simulink model "mrsDiffDrivePathFollowingModel"  (R2023a)
settings: Solver=VariableStepAuto  StartTime=0.0  StopTime=42  FixedStep=0.01  RelTol=1e-3  EnableMultiTasking=on
PreLoadFcn:
  | % Simulation parameters
  | sampleTime = 0.1;
  | 
  | % Vehicle parameters
  | R = 0.1;
  | L = 0.5;
  | 
  | % Lidar parameters
  | load exampleMap
  | scanAngles = linspace(-pi/2,pi/2,51);
  | scanMaxRange = 5;
  | scanSensorOffset = [0,0];
libraries: mobileRoboticsLib x4, simulink x2, robotalgslib x2
settings Model: Creator=scastro  LastModifiedBy=John_117
settings SolverCC: AlgebraicLoopSolver=TrustRegion
settings DataIOCC: LimitDataPoints=on  ReturnWorkspaceOutputs=off
settings OptimizationCC: LifeSpan=inf
settings DebuggingCC: UnconnectedInputMsg=warning  UnconnectedOutputMsg=warning  UnconnectedLineMsg=warning  AllowSymbolicDim=off  SFUnexpectedBacktrackingDiag=warning  SFNoUnconditionalDefaultTransitionDiag=warning  SFExecutionAtInitializationDiag=none  ArithmeticOperatorsInVariantConditions=warning
settings ModelReferenceCC: EnableRefExpFcnMdlSchedulingChecks=on
settings SFSimCC: SimUseLocalCustomCode=off  CustomCodeUndefinedFunction=UseInterfaceOnly
settings RTWCC: RTWUseLocalCustomCode=off
settings CodeAppCC: StateflowObjectComments=on
settings GRTTargetCC: TargetLangStandard=C89/C90 (ANSI)
settings ConfigComp: CovMetricSettings=dw  CovSaveCumulativeToWorkspaceVar=on  CovSaveSingleToWorkspaceVar=on  CovExternalEMLEnable=off  CovSFcnEnable=off
settings SimscapeCC: SimscapeNominalValues="[{\"value\":\"10\",\"unit\":\"V\"},{\"value\":\"1\",\"unit\":\"A\"},{\"value\":\"10\",\"unit\":\"N*m\"},{\"value\":\"10\",\"unit\":\"bar\"},{\"value\":\"100\",\"unit\":\"kJ/kg\"},{\"value\":\"1\",\"unit\":\"kW\"},{\"value\":\"300\",\"unit\":\"K\"},{\"value\":\"100\",\"unit\":\"cm^3/s\"},{\"value\":\"1\",\"unit\":\"kN\"},{\"value\":\"1\",\"unit\":\"g/cm^3\"},{\"value\":\"1\",\"unit\":\"l\"},{\"value\":\"1\",\"unit\":\"cm^2\"},{\"value\":\"60\",\"unit\":\"Hz\"}]"  SimscapeLogType=all  SimscapeLogDataHistory=10000
settings ConfigurationSet: Description=SimMechanics 2G
settings ExplorerConfigSet: InternalSimMechanicsExplorerSettings="<ExplorerConfiguration><canonicalview>default</canonicalview><AnimationSetting><BasePlaybackSpeed>1.0</BasePlaybackSpeed><PlaybackSpeedFactor>1.0</PlaybackSpeedFactor></AnimationSetting><TilePanel><TileInfo><Tiles Columns=\"1\" Count=\"1\" Rows=\"1\"><Column Weight=\"1\"/><Row Weight=\"1\"/><Tile Height=\"1\" Width=\"1\" X=\"0\" Y=\"0\"/></Tiles></TileInfo><SceneInfo><SceneViewer><BGColor><R>0.60000002384185791</R><G>0.60000002384185791</G><B>0.60000002384185791</B></BGColor><Camera><DoPerspective>off</DoPerspective><Position><X>-1.70656042355848525</X><Y>-0.974920623359631922</Y><Z>4.72930454537082046</Z></Position><Center><X>0.552860638431633689</X><Y>1.42025063411503494</Y><Z>1.4843509506914252</Z></Center><Up><X>0.664249622453917166</X><Y>0.300615402055903091</Y><Z>0.684399604848363485</Z></Up><ViewLimDist>1</ViewLimDist><YLim>2.77881717169207398</YLim><XLim>3.55928742670435394</XLim></Camera></SceneViewer></SceneInfo></TilePanel><MechEditorPanel><Cameras/><GfxPanelCameraMap/><VideoCreator><PlaybackSpeedRatio>1.0</PlaybackSpeedRatio><FrameRate>30</FrameRate><VideoFormat>Motion JPEG AVI</VideoFormat><FrameSize>auto</FrameSize></VideoCreator></MechEditorPanel></ExplorerConfiguration>"

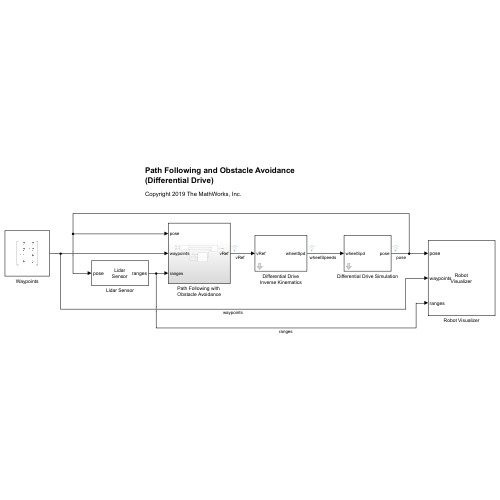
[thumbnail: Simulink's stored preview of the top-level diagram]
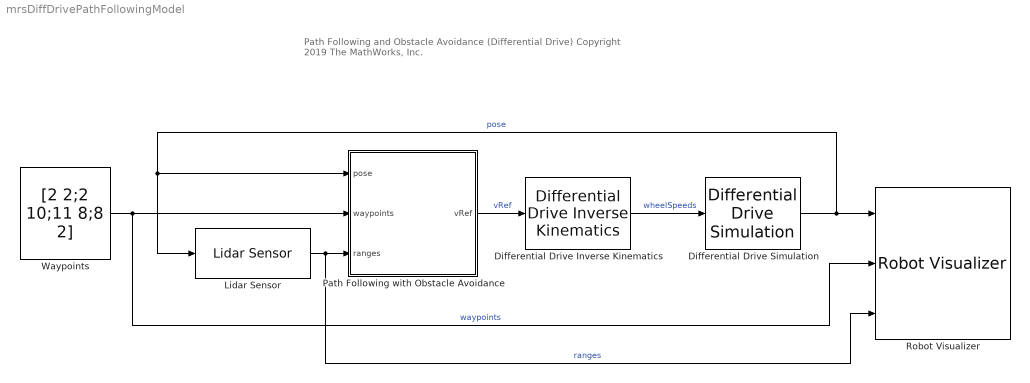
== system mrsDiffDrivePathFollowingModel ==
  note: Path Following and Obstacle Avoidance
      | (Differential Drive)
      |
      | Copyright 2019 The MathWorks, Inc.
  Differential Drive Inverse Kinematics : mobileRoboticsLib/Kinematic Models/Differential Drive/Differential Drive Inverse Kinematics  wheelRadius=R  wheelBase=L
      settings: SourceProductName=Mobile Robotics Simulation Toolbox
  Differential Drive Simulation : mobileRoboticsLib/Kinematic Models/Differential Drive/Differential Drive Simulation  wheelRadius=R  wheelBase=L  initX=2  initY=2  initAngle=0  Ts=sampleTime
      settings: SourceProductName=Mobile Robotics Simulation Toolbox
  Lidar Sensor : mobileRoboticsLib/Environments/Lidar Sensor  mapName=map  sensorOffset=scanSensorOffset  scanAngles=scanAngles  maxRange=scanMaxRange
      settings: SourceProductName=Mobile Robotics Simulation Toolbox
  Path Following with Obstacle Avoidance : Subsystem
  Robot Visualizer : mobileRoboticsLib/Environments/Robot Visualizer  Priority=99  robotRadius=0  mapName=map  showTrajectory=on  hasWaypoints=on  hasLidar=on  sensorOffset=scanSensorOffset  scanAngles=scanAngles  hasObjDetector=off  objDetectorOffset=[ 0, 0 ]  objDetectorAngle=0  objDetectorFOV=0  objDetectorMaxRange=0  objectColors=0  objectMarkers='s'
  Waypoints : Constant  Value=[2 2;2 10;11 8;8 2]
  wires:
  Differential Drive Simulation/1 -> Robot Visualizer/1, Path Following with Obstacle Avoidance/1(pose), Lidar Sensor/1  "pose"
  Differential Drive Inverse Kinematics/1 -> Differential Drive Simulation/1  "wheelSpeeds"
  Waypoints/1 -> Path Following with Obstacle Avoidance/2(waypoints), Robot Visualizer/2  "waypoints"
  Path Following with Obstacle Avoidance/1(vRef) -> Differential Drive Inverse Kinematics/1  "vRef"
  Lidar Sensor/1 -> Robot Visualizer/3, Path Following with Obstacle Avoidance/3(ranges)  "ranges"

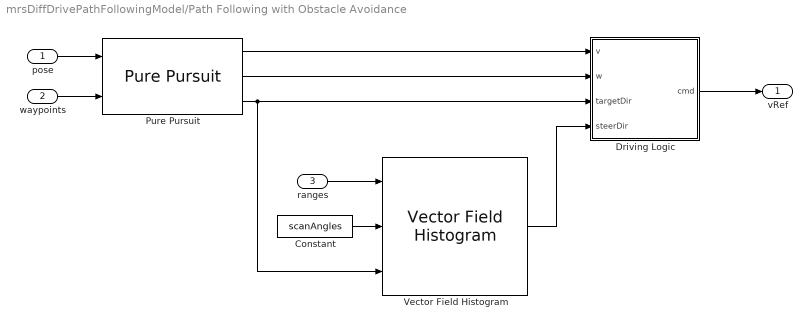
== system mrsDiffDrivePathFollowingModel/Path Following with Obstacle Avoidance ==
  pose : Inport
  waypoints : Inport  Port=2
  ranges : Inport  Port=3
  Constant : Constant  Value=scanAngles
  Driving Logic : Subsystem
  Pure Pursuit : robotalgslib/Pure Pursuit  DesiredLinearVelocity=0.75  MaxAngularVelocity=1.5  LookaheadDistance=0.5  TargetDirPort=on  SimulateUsing=Interpreted execution
  Vector Field Histogram : robotalgslib/Vector Field Histogram  NumAngularSectors=36  DistanceLimits=[ 0.05, 3 ]  HistogramThresholds=[ 5, 10 ]  RobotRadius=L  SafetyDistance=L  MinTurningRadius=0.25  SimulateUsing=Interpreted execution  TargetDirectionWeight=5  CurrentDirectionWeight=2  PreviousDirectionWeight=2
  vRef : Outport  VectorParamsAs1DForOutWhenUnconnected=off
  wires:
  pose/1 -> Pure Pursuit/1
  Pure Pursuit/3 -> Driving Logic/3(targetDir), Vector Field Histogram/3
  Pure Pursuit/1 -> Driving Logic/1(v)
  Constant/1 -> Vector Field Histogram/2
  Vector Field Histogram/1 -> Driving Logic/4(steerDir)
  ranges/1 -> Vector Field Histogram/1
  waypoints/1 -> Pure Pursuit/2
  Pure Pursuit/2 -> Driving Logic/2(w)
  Driving Logic/1(cmd) -> vRef/1

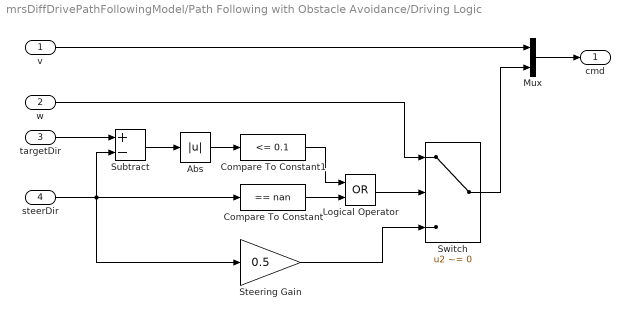
== system mrsDiffDrivePathFollowingModel/Path Following with Obstacle Avoidance/Driving Logic ==
  v : Inport
  w : Inport  Port=2
  targetDir : Inport  Port=3
  steerDir : Inport  Port=4
  Abs : Abs  SaturateOnIntegerOverflow=off
  Compare To Constant : simulink/Logic and Bit Operations/Compare To Constant  relop===  const=nan  OutDataTypeStr=boolean
  Compare To Constant1 : simulink/Logic and Bit Operations/Compare To Constant  relop=<=  const=0.1  OutDataTypeStr=boolean
  Logical Operator : Logic  Operator=OR  AllPortsSameDT=off  OutDataTypeStr=boolean
  Mux : Mux  Inputs=2
  Steering Gain : Gain  Gain=0.5
  Subtract : Sum  Inputs=+-
  Switch : Switch  Criteria=u2 ~= 0  SaturateOnIntegerOverflow=off  InputSameDT=off
  cmd : Outport  VectorParamsAs1DForOutWhenUnconnected=off
  wires:
  v/1 -> Mux/1
  steerDir/1 -> Steering Gain/1, Subtract/2, Compare To Constant/1
  Compare To Constant/1 -> Logical Operator/2
  targetDir/1 -> Subtract/1
  Subtract/1 -> Abs/1
  Abs/1 -> Compare To Constant1/1
  Compare To Constant1/1 -> Logical Operator/1
  Mux/1 -> cmd/1
  Logical Operator/1 -> Switch/2
  w/1 -> Switch/1
  Switch/1 -> Mux/2
  Steering Gain/1 -> Switch/3
